simulink library "see_saw_mario"  (R2013b)
settings: Solver=ode45  StartTime=0.0  StopTime=10.0  RelTol=1e-3
undefined symbols (not defined in the file): DiscIntNeverNeededParam, K, R
libraries: legonxtlib x7, simulink x4, see_saw_mario x2
settings Model: Creator=mbiesiad  LastModifiedBy=pvinnako

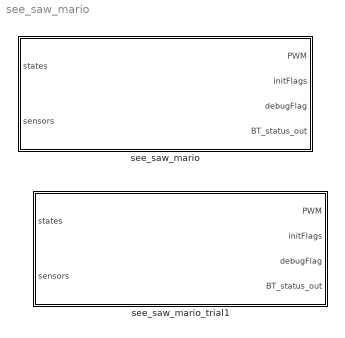
== system see_saw_mario ==
  see_saw_mario : Stateflow chart  TreatAsAtomicUnit=on
  see_saw_mario_trial1 : Stateflow chart  TreatAsAtomicUnit=on

== system see_saw_mario/see_saw_mario/see_saw_mode.DispVar ==
  Var : Inport  OutDataTypeStr=single  PortDimensions=1
  f : TriggerPort  TriggerType=function-call
      settings: CopyFcn=Stateflow.SLINSF.SimulinkMan.removeBlockPreDeleteFcn  PreDeleteFcn=Stateflow.SLINSF.SimulinkMan.unsafePredeleteFcn
  Gain : Gain  Gain=100
  LCD : legonxtlib/LCD  slcdStr=Light  slcdLine=2  slcdFormat=Decimal
  wires:
  Gain/1 -> LCD/1
  Var/1 -> Gain/1

== system see_saw_mario/see_saw_mario/see_saw_mode.Speak ==
  f : TriggerPort  TriggerType=function-call
      settings: CopyFcn=Stateflow.SLINSF.SimulinkMan.removeBlockPreDeleteFcn  PreDeleteFcn=Stateflow.SLINSF.SimulinkMan.unsafePredeleteFcn
  Constant : Constant  Value=50
  Speaker : legonxtlib/Speaker  sinputMode=Volume only  sspeakerFreq=800  sspeakerVolume=50  sspeakerDuration=100
  wires:
  Constant/1 -> Speaker/1

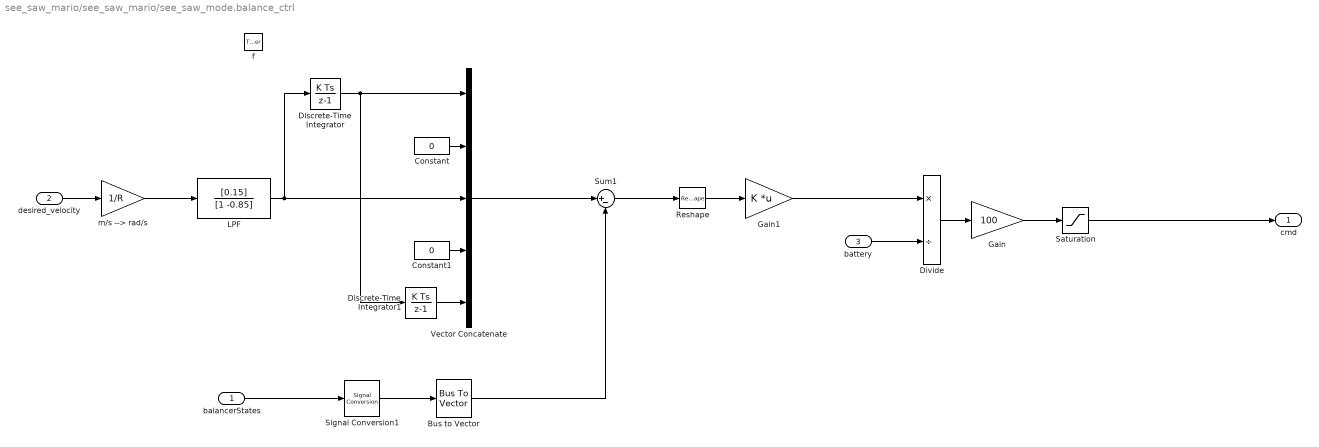
== system see_saw_mario/see_saw_mario/see_saw_mode.balance_ctrl ==
  balancerStates : Inport  OutDataTypeStr=Bus: Balancer_States_Bus  PortDimensions=1
  desired_velocity : Inport  Port=2  OutDataTypeStr=single  PortDimensions=1  BusOutputAsStruct=on
  battery : Inport  Port=3  OutDataTypeStr=double  PortDimensions=1
  f : TriggerPort  TriggerType=function-call
      settings: CopyFcn=Stateflow.SLINSF.SimulinkMan.removeBlockPreDeleteFcn  PreDeleteFcn=Stateflow.SLINSF.SimulinkMan.unsafePredeleteFcn
  Bus to Vector : BusToVector
  Constant : Constant  Value=0  OutDataTypeStr=single
  Constant1 : Constant  Value=0  OutDataTypeStr=single
  Discrete-Time Integrator : DiscreteIntegrator  SampleTime=-1  ICPrevOutput=DiscIntNeverNeededParam  ICPrevScaledInput=DiscIntNeverNeededParam
  Discrete-Time Integrator1 : DiscreteIntegrator  SampleTime=-1  ICPrevOutput=DiscIntNeverNeededParam  ICPrevScaledInput=DiscIntNeverNeededParam
  Divide : Product  Inputs=*/
  Gain : Gain  Gain=100
  Gain1 : Gain  Gain=K  Multiplication=Matrix(K*u)
  LPF : DiscreteFilter  Numerator=[0.15]  Denominator=[1 -0.85]
  Reshape : Reshape  OutputDimensionality=Column vector (2-D)
  Saturation : Saturate  UpperLimit=100  LowerLimit=-100  OutDataTypeStr=single
  Signal Conversion1 : SignalConversion  ConversionOutput=Virtual bus
  Sum1 : Sum  Inputs=|+-
  Vector Concatenate : Concatenate  NumInputs=5
  m/s --> rad/s : Gain  Gain=1/R
  cmd : Outport  OutDataTypeStr=single  PortDimensions=1  InitialOutput=0
  wires:
  Discrete-Time Integrator1/1 -> Vector Concatenate/5
  Discrete-Time Integrator/1 -> Vector Concatenate/1, Discrete-Time Integrator1/1
  Constant1/1 -> Vector Concatenate/4
  LPF/1 -> Vector Concatenate/3, Discrete-Time Integrator/1
  Constant/1 -> Vector Concatenate/2
  m/s --> rad/s/1 -> LPF/1
  Signal Conversion1/1 -> Bus to Vector/1
  Divide/1 -> Gain/1
  Gain/1 -> Saturation/1
  Gain1/1 -> Divide/1
  Saturation/1 -> cmd/1
  battery/1 -> Divide/2
  Vector Concatenate/1 -> Sum1/1
  balancerStates/1 -> Signal Conversion1/1
  Bus to Vector/1 -> Sum1/2
  desired_velocity/1 -> m/s --> rad/s/1
  Sum1/1 -> Reshape/1
  Reshape/1 -> Gain1/1

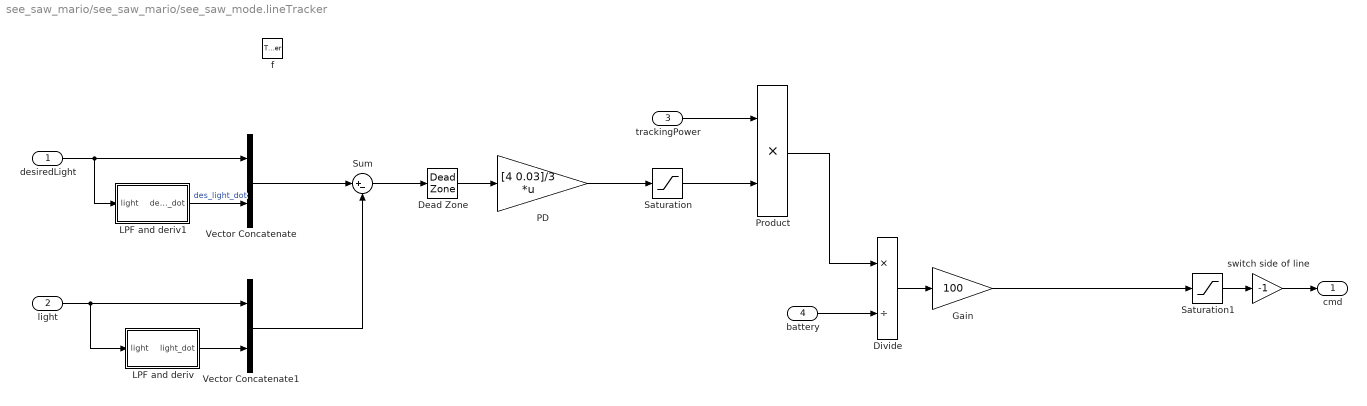
== system see_saw_mario/see_saw_mario/see_saw_mode.lineTracker ==
  desiredLight : Inport  OutDataTypeStr=single  PortDimensions=1
  light : Inport  Port=2  OutDataTypeStr=single  PortDimensions=1
  trackingPower : Inport  Port=3  OutDataTypeStr=single  PortDimensions=1
  battery : Inport  Port=4  OutDataTypeStr=double  PortDimensions=1
  f : TriggerPort  TriggerType=function-call
      settings: CopyFcn=Stateflow.SLINSF.SimulinkMan.removeBlockPreDeleteFcn  PreDeleteFcn=Stateflow.SLINSF.SimulinkMan.unsafePredeleteFcn
  Dead Zone : DeadZone  LowerValue=-0.02  UpperValue=0.02  SaturateOnIntegerOverflow=on
  Divide : Product  Inputs=*/
  Gain : Gain  Gain=100
  LPF and deriv : Subsystem
  LPF and deriv1 : Subsystem
  PD : Gain  Gain="[4  0.03]/3"  Multiplication=Matrix(K*u)
  Product : Product
  Saturation : Saturate  UpperLimit=6  LowerLimit=-6
  Saturation1 : Saturate  UpperLimit=100  LowerLimit=-100  OutDataTypeStr=single
  Sum : Sum  Inputs=|+-
  Vector Concatenate : Concatenate
  Vector Concatenate1 : Concatenate
  switch side of line : Gain  Gain=-1
  cmd : Outport  OutDataTypeStr=single  PortDimensions=1
  wires:
  Divide/1 -> Gain/1
  Gain/1 -> Saturation1/1
  battery/1 -> Divide/2
  Saturation1/1 -> switch side of line/1
  Product/1 -> Divide/1
  trackingPower/1 -> Product/1
  Saturation/1 -> Product/2
  PD/1 -> Saturation/1
  Dead Zone/1 -> PD/1
  Sum/1 -> Dead Zone/1
  Vector Concatenate1/1 -> Sum/2
  Vector Concatenate/1 -> Sum/1
  light/1 -> Vector Concatenate1/1, LPF and deriv/1(light)
  LPF and deriv/1(light_dot) -> Vector Concatenate1/2
  LPF and deriv1/1(des_light_dot) -> Vector Concatenate/2  "des_light_dot"
  desiredLight/1 -> LPF and deriv1/1(light), Vector Concatenate/1
  switch side of line/1 -> cmd/1

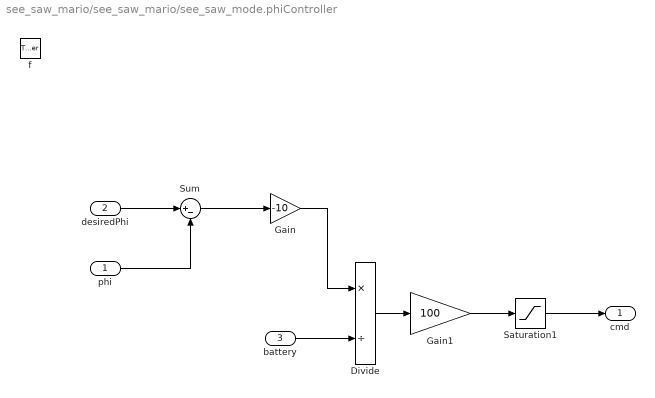
== system see_saw_mario/see_saw_mario/see_saw_mode.phiController ==
  phi : Inport  OutDataTypeStr=single  PortDimensions=1
  desiredPhi : Inport  Port=2  OutDataTypeStr=single  PortDimensions=1
  battery : Inport  Port=3  OutDataTypeStr=double  PortDimensions=1
  f : TriggerPort  TriggerType=function-call
      settings: CopyFcn=Stateflow.SLINSF.SimulinkMan.removeBlockPreDeleteFcn  PreDeleteFcn=Stateflow.SLINSF.SimulinkMan.unsafePredeleteFcn
  Divide : Product  Inputs=*/
  Gain : Gain  Gain=-10
  Gain1 : Gain  Gain=100
  Saturation1 : Saturate  UpperLimit=100  LowerLimit=-100  OutDataTypeStr=single
  Sum : Sum  Inputs=|+-
  cmd : Outport
  wires:
  Saturation1/1 -> cmd/1
  Gain/1 -> Divide/1
  Divide/1 -> Gain1/1
  Gain1/1 -> Saturation1/1
  battery/1 -> Divide/2
  Sum/1 -> Gain/1
  phi/1 -> Sum/2
  desiredPhi/1 -> Sum/1

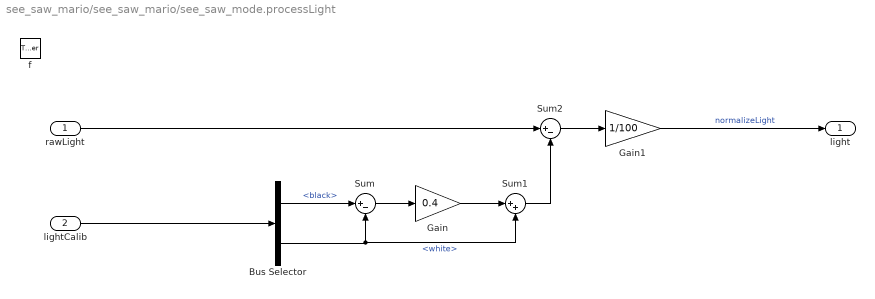
== system see_saw_mario/see_saw_mario/see_saw_mode.processLight ==
  rawLight : Inport  OutDataTypeStr=single  PortDimensions=1
  lightCalib : Inport  Port=2  OutDataTypeStr=Bus: Light_Bus  PortDimensions=1
  f : TriggerPort  TriggerType=function-call
      settings: CopyFcn=Stateflow.SLINSF.SimulinkMan.removeBlockPreDeleteFcn  PreDeleteFcn=Stateflow.SLINSF.SimulinkMan.unsafePredeleteFcn
  Bus Selector : BusSelector  OutputSignals=black,white
  Gain : Gain  Gain=0.4
  Gain1 : Gain  Gain=1/100
  Sum : Sum  Inputs=|+-
  Sum1 : Sum  Inputs=|++
  Sum2 : Sum  Inputs=|+-
  light : Outport
  wires:
  Gain1/1 -> light/1  "normalizeLight"
  Sum2/1 -> Gain1/1
  Sum1/1 -> Sum2/2
  rawLight/1 -> Sum2/1
  Gain/1 -> Sum1/1
  Sum/1 -> Gain/1
  Bus Selector/2 -> Sum/2, Sum1/2  "<white>"
  Bus Selector/1 -> Sum/1  "<black>"
  lightCalib/1 -> Bus Selector/1

== system see_saw_mario/see_saw_mario/see_saw_mode.tail_controller ==
  note: Could be improved, PI for example
  current : Inport  OutDataTypeStr=single  PortDimensions=1
  desired : Inport  Port=2  OutDataTypeStr=single  PortDimensions=1
  f : TriggerPort  TriggerType=function-call
      settings: CopyFcn=Stateflow.SLINSF.SimulinkMan.removeBlockPreDeleteFcn  PreDeleteFcn=Stateflow.SLINSF.SimulinkMan.unsafePredeleteFcn
  Gain : Gain  Gain=250
  Saturation : Saturate  UpperLimit=100  LowerLimit=-100  OutDataTypeStr=single
  Sum : Sum  Inputs=|+-
  cmd : Outport  OutDataTypeStr=single  PortDimensions=1  InitialOutput=0
  wires:
  Saturation/1 -> cmd/1
  Gain/1 -> Saturation/1
  desired/1 -> Sum/1
  current/1 -> Sum/2
  Sum/1 -> Gain/1

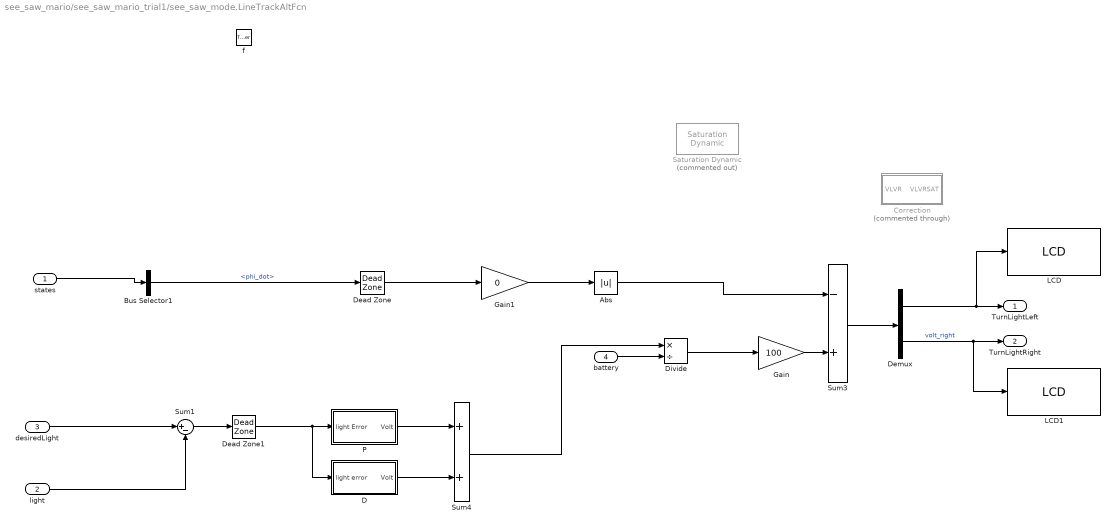
== system see_saw_mario/see_saw_mario_trial1/see_saw_mode.LineTrackAltFcn ==
  states : Inport  OutDataTypeStr=Bus: States_Bus  PortDimensions=1
  light : Inport  Port=2  OutDataTypeStr=single  PortDimensions=1
  desiredLight : Inport  Port=3  OutDataTypeStr=single  PortDimensions=1
  battery : Inport  Port=4  OutDataTypeStr=single  PortDimensions=1
  f : TriggerPort  TriggerType=function-call
      settings: CopyFcn=Stateflow.SLINSF.SimulinkMan.removeBlockPreDeleteFcn  PreDeleteFcn=Stateflow.SLINSF.SimulinkMan.unsafePredeleteFcn
  Abs : Abs
  Bus Selector1 : BusSelector  OutputSignals=phi_dot
  Correction : Subsystem  Commented=through
  D : Subsystem
  Dead Zone : DeadZone  LowerValue=-3  UpperValue=3  SaturateOnIntegerOverflow=on
  Dead Zone1 : DeadZone  LowerValue=0  UpperValue=0  SaturateOnIntegerOverflow=on
  Demux : Demux  Outputs=2
  Divide : Product  Inputs=*/
  Gain : Gain  Gain=100
  Gain1 : Gain  Gain=0
  LCD : legonxtlib/LCD  slcdStr=TurnL  slcdLine=5  slcdFormat=Decimal
  LCD1 : legonxtlib/LCD  slcdStr=TurnR  slcdLine=6  slcdFormat=Decimal
  P : Subsystem
  Saturation Dynamic : simulink/Discontinuities/Saturation Dynamic  Commented=on  OutMin=[]  OutMax=[]  OutDataTypeStr=Inherit: Same as second input  OutDataType=fixdt(1, 16)  OutScaling=2^-10  DoSatur=off
  Sum1 : Sum  Inputs=|+-
  Sum3 : Sum  Inputs=-+
  Sum4 : Sum
  TurnLightLeft : Outport  OutDataTypeStr=single  InitialOutput=0
  TurnLightRight : Outport  Port=2  OutDataTypeStr=single  InitialOutput=0
  wires:
  Dead Zone1/1 -> D/1(light error), P/1(light Error)
  Dead Zone/1 -> Gain1/1
  Demux/2 -> LCD1/1, TurnLightRight/1  "volt_right"
  Demux/1 -> LCD/1, TurnLightLeft/1
  light/1 -> Sum1/2
  Sum1/1 -> Dead Zone1/1
  states/1 -> Bus Selector1/1
  desiredLight/1 -> Sum1/1
  P/1(Volt) -> Sum4/1
  D/1(Volt) -> Sum4/2
  Gain/1 -> Sum3/2
  Abs/1 -> Sum3/1
  Gain1/1 -> Abs/1
  Bus Selector1/1 -> Dead Zone/1  "<phi_dot>"
  Sum3/1 -> Demux/1
  battery/1 -> Divide/2
  Divide/1 -> Gain/1
  Sum4/1 -> Divide/1

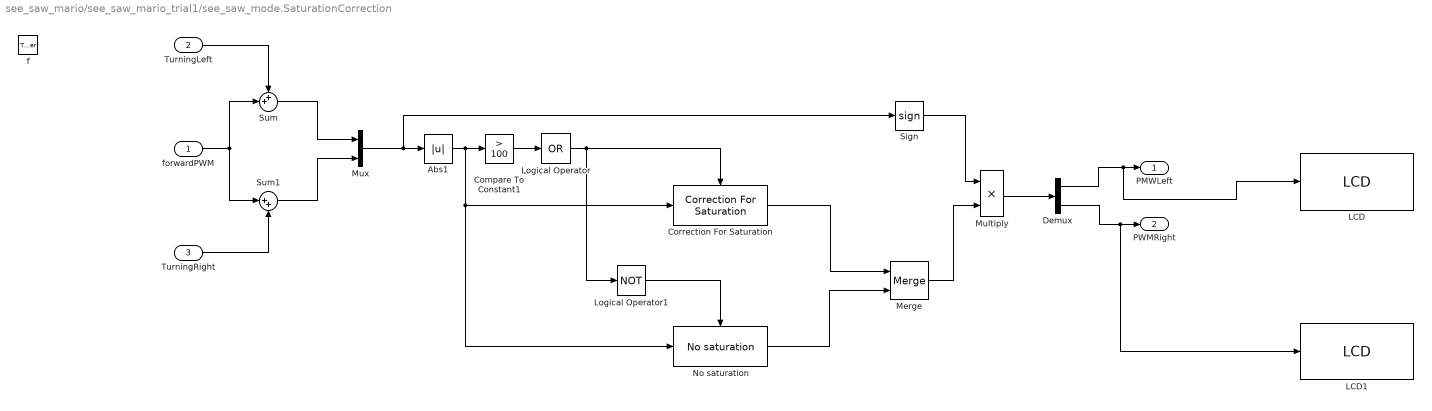
== system see_saw_mario/see_saw_mario_trial1/see_saw_mode.SaturationCorrection ==
  forwardPWM : Inport  OutDataTypeStr=single  PortDimensions=1
  TurningLeft : Inport  Port=2  OutDataTypeStr=single  PortDimensions=1
  TurningRight : Inport  Port=3  OutDataTypeStr=single  PortDimensions=1
  f : TriggerPort  TriggerType=function-call
      settings: CopyFcn=Stateflow.SLINSF.SimulinkMan.removeBlockPreDeleteFcn  PreDeleteFcn=Stateflow.SLINSF.SimulinkMan.unsafePredeleteFcn
  Abs1 : Abs
  Compare To Constant1 : simulink/Logic and Bit Operations/Compare To Constant  relop=>  const=100  OutDataTypeStr=boolean
  Correction For Saturation : see_saw_mario/see_saw_mario/see_saw_mode.LineTrackAltFcn/Correction/Correction For Saturation
  Demux : Demux  Outputs=2
  LCD : legonxtlib/LCD  slcdStr=VL  slcdLine=3  slcdFormat=Decimal
  LCD1 : legonxtlib/LCD  slcdStr=VR  slcdLine=4  slcdFormat=Decimal
  Logical Operator : Logic  Operator=OR  Inputs=1  AllPortsSameDT=off  OutDataTypeStr=boolean
  Logical Operator1 : Logic  Operator=NOT  Inputs=1  AllPortsSameDT=off  OutDataTypeStr=boolean
  Merge : Merge
  Multiply : Product  Inputs=**
  Mux : Mux  Inputs=2
  No saturation : see_saw_mario/see_saw_mario/see_saw_mode.LineTrackAltFcn/Correction/No saturation
  Sign : Signum
  Sum : Sum  Inputs=++|
  Sum1 : Sum  Inputs=|++
  PMWLeft : Outport  OutDataTypeStr=single  PortDimensions=1
  PWMRight : Outport  Port=2  OutDataTypeStr=single  PortDimensions=1
  wires:
  Mux/1 -> Sign/1, Abs1/1
  Abs1/1 -> No saturation/1, Correction For Saturation/1, Compare To Constant1/1
  Compare To Constant1/1 -> Logical Operator/1
  Logical Operator/1 -> Logical Operator1/1, Correction For Saturation/Enable
  Logical Operator1/1 -> No saturation/Enable
  Correction For Saturation/1 -> Merge/1
  No saturation/1 -> Merge/2
  Merge/1 -> Multiply/2
  Sign/1 -> Multiply/1
  Multiply/1 -> Demux/1
  forwardPWM/1 -> Sum1/1, Sum/2
  TurningLeft/1 -> Sum/1
  TurningRight/1 -> Sum1/2
  Sum/1 -> Mux/1
  Sum1/1 -> Mux/2
  Demux/1 -> LCD/1, PMWLeft/1
  Demux/2 -> LCD1/1, PWMRight/1

== system see_saw_mario/see_saw_mario_trial1/see_saw_mode.Speak ==
  f : TriggerPort  TriggerType=function-call
      settings: CopyFcn=Stateflow.SLINSF.SimulinkMan.removeBlockPreDeleteFcn  PreDeleteFcn=Stateflow.SLINSF.SimulinkMan.unsafePredeleteFcn
  Constant : Constant  Value=50
  Speaker : legonxtlib/Speaker  sinputMode=Volume only  sspeakerFreq=800  sspeakerVolume=50  sspeakerDuration=100
  wires:
  Constant/1 -> Speaker/1

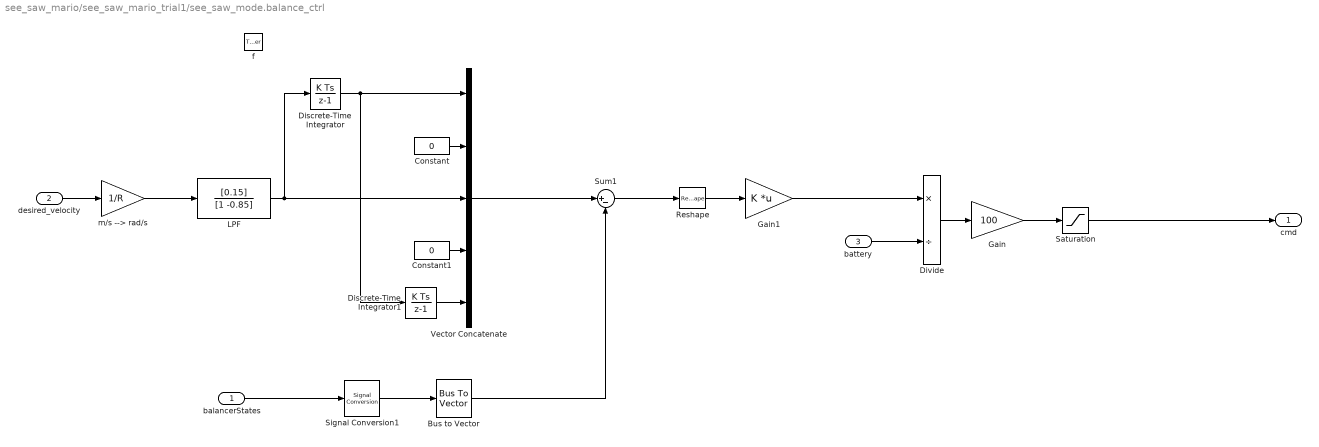
== system see_saw_mario/see_saw_mario_trial1/see_saw_mode.balance_ctrl ==
  balancerStates : Inport  OutDataTypeStr=Bus: Balancer_States_Bus  PortDimensions=1
  desired_velocity : Inport  Port=2  OutDataTypeStr=single  PortDimensions=1  BusOutputAsStruct=on
  battery : Inport  Port=3  OutDataTypeStr=double  PortDimensions=1
  f : TriggerPort  TriggerType=function-call
      settings: CopyFcn=Stateflow.SLINSF.SimulinkMan.removeBlockPreDeleteFcn  PreDeleteFcn=Stateflow.SLINSF.SimulinkMan.unsafePredeleteFcn
  Bus to Vector : BusToVector
  Constant : Constant  Value=0  OutDataTypeStr=single
  Constant1 : Constant  Value=0  OutDataTypeStr=single
  Discrete-Time Integrator : DiscreteIntegrator  SampleTime=-1  ICPrevOutput=DiscIntNeverNeededParam  ICPrevScaledInput=DiscIntNeverNeededParam
  Discrete-Time Integrator1 : DiscreteIntegrator  SampleTime=-1  ICPrevOutput=DiscIntNeverNeededParam  ICPrevScaledInput=DiscIntNeverNeededParam
  Divide : Product  Inputs=*/
  Gain : Gain  Gain=100
  Gain1 : Gain  Gain=K  Multiplication=Matrix(K*u)
  LPF : DiscreteFilter  Numerator=[0.15]  Denominator=[1 -0.85]
  Reshape : Reshape  OutputDimensionality=Column vector (2-D)
  Saturation : Saturate  UpperLimit=100  LowerLimit=-100  OutDataTypeStr=single
  Signal Conversion1 : SignalConversion  ConversionOutput=Virtual bus
  Sum1 : Sum  Inputs=|+-
  Vector Concatenate : Concatenate  NumInputs=5
  m/s --> rad/s : Gain  Gain=1/R
  cmd : Outport  OutDataTypeStr=single  PortDimensions=1  InitialOutput=0
  wires:
  Reshape/1 -> Gain1/1
  Sum1/1 -> Reshape/1
  desired_velocity/1 -> m/s --> rad/s/1
  Bus to Vector/1 -> Sum1/2
  balancerStates/1 -> Signal Conversion1/1
  Vector Concatenate/1 -> Sum1/1
  battery/1 -> Divide/2
  Saturation/1 -> cmd/1
  Gain1/1 -> Divide/1
  Gain/1 -> Saturation/1
  Divide/1 -> Gain/1
  Signal Conversion1/1 -> Bus to Vector/1
  m/s --> rad/s/1 -> LPF/1
  Constant/1 -> Vector Concatenate/2
  LPF/1 -> Discrete-Time Integrator/1, Vector Concatenate/3
  Constant1/1 -> Vector Concatenate/4
  Discrete-Time Integrator/1 -> Discrete-Time Integrator1/1, Vector Concatenate/1
  Discrete-Time Integrator1/1 -> Vector Concatenate/5

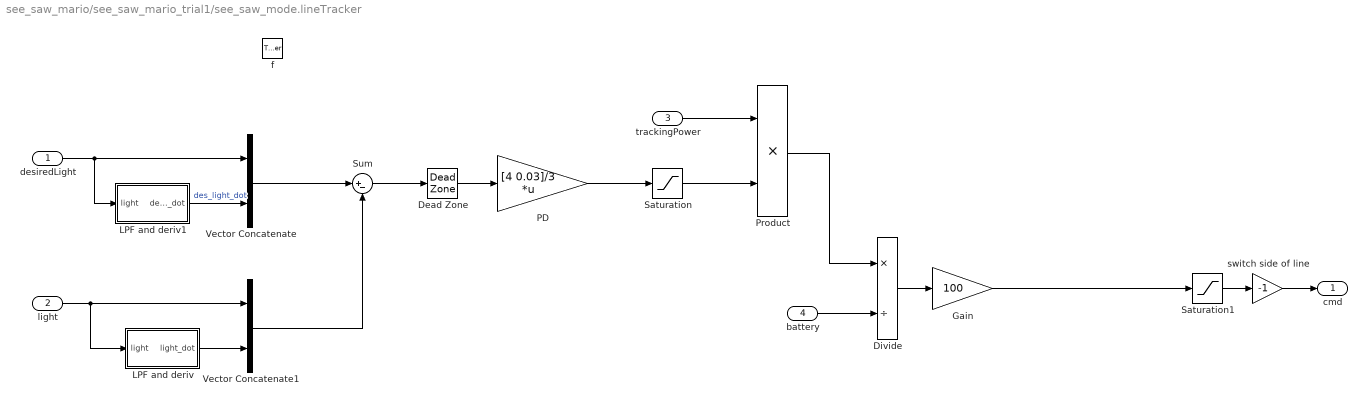
== system see_saw_mario/see_saw_mario_trial1/see_saw_mode.lineTracker ==
  desiredLight : Inport  OutDataTypeStr=single  PortDimensions=1
  light : Inport  Port=2  OutDataTypeStr=single  PortDimensions=1
  trackingPower : Inport  Port=3  OutDataTypeStr=single  PortDimensions=1
  battery : Inport  Port=4  OutDataTypeStr=double  PortDimensions=1
  f : TriggerPort  TriggerType=function-call
      settings: CopyFcn=Stateflow.SLINSF.SimulinkMan.removeBlockPreDeleteFcn  PreDeleteFcn=Stateflow.SLINSF.SimulinkMan.unsafePredeleteFcn
  Dead Zone : DeadZone  LowerValue=-0.02  UpperValue=0.02  SaturateOnIntegerOverflow=on
  Divide : Product  Inputs=*/
  Gain : Gain  Gain=100
  LPF and deriv : Subsystem
  LPF and deriv1 : Subsystem
  PD : Gain  Gain="[4  0.03]/3"  Multiplication=Matrix(K*u)
  Product : Product
  Saturation : Saturate  UpperLimit=6  LowerLimit=-6
  Saturation1 : Saturate  UpperLimit=100  LowerLimit=-100  OutDataTypeStr=single
  Sum : Sum  Inputs=|+-
  Vector Concatenate : Concatenate
  Vector Concatenate1 : Concatenate
  switch side of line : Gain  Gain=-1
  cmd : Outport  OutDataTypeStr=single  PortDimensions=1
  wires:
  switch side of line/1 -> cmd/1
  desiredLight/1 -> Vector Concatenate/1, LPF and deriv1/1(light)
  LPF and deriv1/1(des_light_dot) -> Vector Concatenate/2  "des_light_dot"
  LPF and deriv/1(light_dot) -> Vector Concatenate1/2
  light/1 -> LPF and deriv/1(light), Vector Concatenate1/1
  Vector Concatenate/1 -> Sum/1
  Vector Concatenate1/1 -> Sum/2
  Sum/1 -> Dead Zone/1
  Dead Zone/1 -> PD/1
  PD/1 -> Saturation/1
  Saturation/1 -> Product/2
  trackingPower/1 -> Product/1
  Product/1 -> Divide/1
  Saturation1/1 -> switch side of line/1
  battery/1 -> Divide/2
  Gain/1 -> Saturation1/1
  Divide/1 -> Gain/1

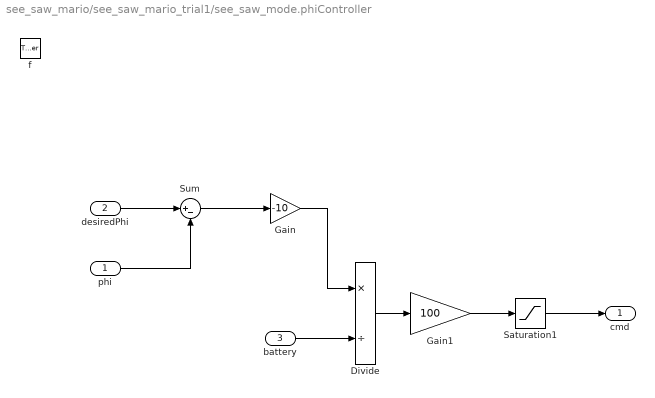
== system see_saw_mario/see_saw_mario_trial1/see_saw_mode.phiController ==
  phi : Inport  OutDataTypeStr=single  PortDimensions=1
  desiredPhi : Inport  Port=2  OutDataTypeStr=single  PortDimensions=1
  battery : Inport  Port=3  OutDataTypeStr=double  PortDimensions=1
  f : TriggerPort  TriggerType=function-call
      settings: CopyFcn=Stateflow.SLINSF.SimulinkMan.removeBlockPreDeleteFcn  PreDeleteFcn=Stateflow.SLINSF.SimulinkMan.unsafePredeleteFcn
  Divide : Product  Inputs=*/
  Gain : Gain  Gain=-10
  Gain1 : Gain  Gain=100
  Saturation1 : Saturate  UpperLimit=100  LowerLimit=-100  OutDataTypeStr=single
  Sum : Sum  Inputs=|+-
  cmd : Outport
  wires:
  desiredPhi/1 -> Sum/1
  phi/1 -> Sum/2
  Sum/1 -> Gain/1
  battery/1 -> Divide/2
  Gain1/1 -> Saturation1/1
  Divide/1 -> Gain1/1
  Gain/1 -> Divide/1
  Saturation1/1 -> cmd/1

== system see_saw_mario/see_saw_mario_trial1/see_saw_mode.processLight ==
  rawLight : Inport  OutDataTypeStr=single  PortDimensions=1
  lightCalib : Inport  Port=2  OutDataTypeStr=Bus: Light_Bus  PortDimensions=1
  f : TriggerPort  TriggerType=function-call
      settings: CopyFcn=Stateflow.SLINSF.SimulinkMan.removeBlockPreDeleteFcn  PreDeleteFcn=Stateflow.SLINSF.SimulinkMan.unsafePredeleteFcn
  Bus Selector : BusSelector  OutputSignals=black,white
  Gain : Gain  Gain=0.3
  Gain1 : Gain  Gain=1/100
  Sum : Sum  Inputs=|+-
  Sum1 : Sum  Inputs=|++
  Sum2 : Sum  Inputs=|+-
  light : Outport
  wires:
  lightCalib/1 -> Bus Selector/1
  Bus Selector/1 -> Sum/1  "<black>"
  Bus Selector/2 -> Sum1/2, Sum/2  "<white>"
  Sum/1 -> Gain/1
  Gain/1 -> Sum1/1
  rawLight/1 -> Sum2/1
  Sum1/1 -> Sum2/2
  Sum2/1 -> Gain1/1
  Gain1/1 -> light/1  "normalizeLight"

== system see_saw_mario/see_saw_mario_trial1/see_saw_mode.tail_controller ==
  note: Could be improved, PI for example
  current : Inport  OutDataTypeStr=single  PortDimensions=1
  desired : Inport  Port=2  OutDataTypeStr=single  PortDimensions=1
  f : TriggerPort  TriggerType=function-call
      settings: CopyFcn=Stateflow.SLINSF.SimulinkMan.removeBlockPreDeleteFcn  PreDeleteFcn=Stateflow.SLINSF.SimulinkMan.unsafePredeleteFcn
  Gain : Gain  Gain=250
  Saturation : Saturate  UpperLimit=100  LowerLimit=-100  OutDataTypeStr=single
  Sum : Sum  Inputs=|+-
  cmd : Outport  OutDataTypeStr=single  PortDimensions=1  InitialOutput=0
  wires:
  Sum/1 -> Gain/1
  current/1 -> Sum/2
  desired/1 -> Sum/1
  Gain/1 -> Saturation/1
  Saturation/1 -> cmd/1

== system see_saw_mario/see_saw_mario/see_saw_mode.lineTracker/LPF and deriv ==
  light : Inport
  Discrete Filter : DiscreteFilter  Numerator=[0.05]  Denominator=[1 -0.95]
  Gain : Gain  Gain=1/0.004
  Sum3 : Sum  Inputs=+-
  Unit Delay : UnitDelay  SampleTime=-1
  light_dot : Outport
  wires:
  Unit Delay/1 -> Sum3/2
  Gain/1 -> Unit Delay/1, Sum3/1
  Sum3/1 -> light_dot/1  "light_dot"
  Discrete Filter/1 -> Gain/1
  light/1 -> Discrete Filter/1

== system see_saw_mario/see_saw_mario/see_saw_mode.lineTracker/LPF and deriv1 ==
  light : Inport
  Discrete Filter : DiscreteFilter  Numerator=[0.05]  Denominator=[1 -0.95]
  Gain : Gain  Gain=1/0.004
  Sum3 : Sum  Inputs=+-
  Unit Delay : UnitDelay  SampleTime=-1
  des_light_dot : Outport
  wires:
  light/1 -> Discrete Filter/1
  Discrete Filter/1 -> Gain/1
  Sum3/1 -> des_light_dot/1  "des_light_dot"
  Gain/1 -> Sum3/1, Unit Delay/1
  Unit Delay/1 -> Sum3/2

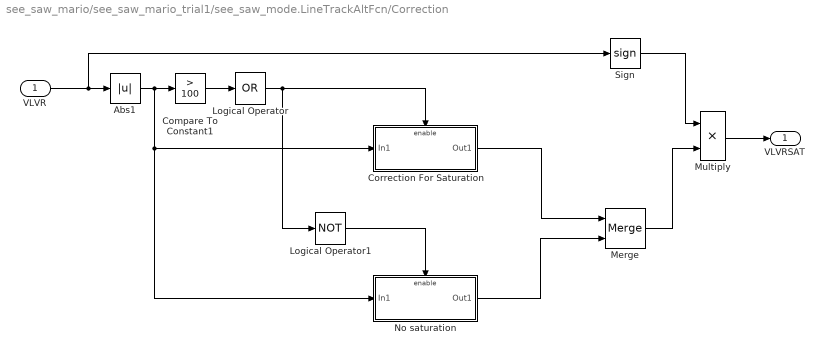
== system see_saw_mario/see_saw_mario_trial1/see_saw_mode.LineTrackAltFcn/Correction ==
  VLVR : Inport
  Abs1 : Abs
  Compare To Constant1 : simulink/Logic and Bit Operations/Compare To Constant  relop=>  const=100  OutDataTypeStr=boolean
  Correction For Saturation : Subsystem  TreatAsAtomicUnit=on
  Logical Operator : Logic  Operator=OR  Inputs=1  AllPortsSameDT=off  OutDataTypeStr=boolean
  Logical Operator1 : Logic  Operator=NOT  Inputs=1  AllPortsSameDT=off  OutDataTypeStr=boolean
  Merge : Merge
  Multiply : Product  Inputs=**
  No saturation : Subsystem  TreatAsAtomicUnit=on
  Sign : Signum
  VLVRSAT : Outport
  wires:
  VLVR/1 -> Sign/1, Abs1/1
  Abs1/1 -> No saturation/1(In1), Correction For Saturation/1(In1), Compare To Constant1/1
  Compare To Constant1/1 -> Logical Operator/1
  Logical Operator/1 -> Logical Operator1/1, Correction For Saturation/Enable
  Logical Operator1/1 -> No saturation/Enable
  Correction For Saturation/1(Out1) -> Merge/1
  No saturation/1(Out1) -> Merge/2
  Merge/1 -> Multiply/2
  Sign/1 -> Multiply/1
  Multiply/1 -> VLVRSAT/1

== system see_saw_mario/see_saw_mario_trial1/see_saw_mode.LineTrackAltFcn/D ==
  light error : Inport
  Abs1 : Abs
  Constant4 : Constant  Value=[3 0]  OutDataTypeStr=single
  Constant5 : Constant  Value=[0 1]  OutDataTypeStr=single
  Discrete Derivative1 : simulink/Discrete/Discrete Derivative  gainval=1.0  ICPrevScaledInput=0.0  InputProcessing=Inherited  OutMin=[]  OutMax=[]  OutDataTypeStr=single  OutputDataTypeScalingMode=single  OutDataType=fixdt(1, 16)  OutScaling=2^-10  DoSatur=off
  Gain2 : Gain  Gain=0.002*10*3
  Low Pass Filter1 : DiscreteFilter  Numerator=[.2]  Denominator=[1 -0.8]
  Product1 : Product  RndMeth=Zero
  Switch1 : Switch
  Volt : Outport
  wires:
  light error/1 -> Low Pass Filter1/1
  Low Pass Filter1/1 -> Discrete Derivative1/1
  Abs1/1 -> Gain2/1
  Constant5/1 -> Switch1/3
  Constant4/1 -> Switch1/1
  Discrete Derivative1/1 -> Switch1/2, Abs1/1
  Switch1/1 -> Product1/1
  Gain2/1 -> Product1/2
  Product1/1 -> Volt/1

== system see_saw_mario/see_saw_mario_trial1/see_saw_mode.LineTrackAltFcn/P ==
  light Error : Inport
  Abs : Abs
  Constant2 : Constant  Value=[3 0]  OutDataTypeStr=single
  Constant3 : Constant  Value=[0 1]  OutDataTypeStr=single
  Gain4 : Gain  Gain=0.05*10*3
  Product : Product  RndMeth=Zero
  Switch : Switch
  Volt : Outport
  wires:
  light Error/1 -> Abs/1, Switch/2
  Switch/1 -> Product/1
  Constant3/1 -> Switch/3
  Constant2/1 -> Switch/1
  Abs/1 -> Gain4/1
  Gain4/1 -> Product/2
  Product/1 -> Volt/1

== system see_saw_mario/see_saw_mario_trial1/see_saw_mode.lineTracker/LPF and deriv ==
  light : Inport
  Discrete Filter : DiscreteFilter  Numerator=[0.05]  Denominator=[1 -0.95]
  Gain : Gain  Gain=1/0.004
  Sum3 : Sum  Inputs=+-
  Unit Delay : UnitDelay  SampleTime=-1
  light_dot : Outport
  wires:
  light/1 -> Discrete Filter/1
  Discrete Filter/1 -> Gain/1
  Sum3/1 -> light_dot/1  "light_dot"
  Gain/1 -> Sum3/1, Unit Delay/1
  Unit Delay/1 -> Sum3/2

== system see_saw_mario/see_saw_mario_trial1/see_saw_mode.lineTracker/LPF and deriv1 ==
  light : Inport
  Discrete Filter : DiscreteFilter  Numerator=[0.05]  Denominator=[1 -0.95]
  Gain : Gain  Gain=1/0.004
  Sum3 : Sum  Inputs=+-
  Unit Delay : UnitDelay  SampleTime=-1
  des_light_dot : Outport
  wires:
  Unit Delay/1 -> Sum3/2
  Gain/1 -> Unit Delay/1, Sum3/1
  Sum3/1 -> des_light_dot/1  "des_light_dot"
  Discrete Filter/1 -> Gain/1
  light/1 -> Discrete Filter/1

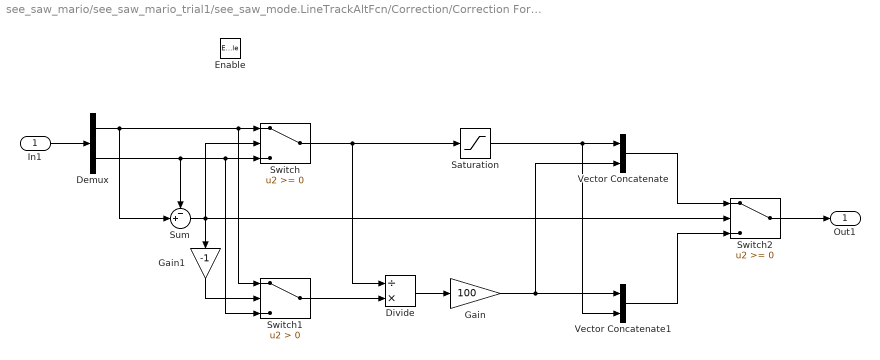
== system see_saw_mario/see_saw_mario_trial1/see_saw_mode.LineTrackAltFcn/Correction/Correction For Saturation ==
  In1 : Inport
  Enable : EnablePort
  Demux : Demux  Outputs=2
  Divide : Product  Inputs=/*
  Gain : Gain  Gain=100
  Gain1 : Gain  Gain=-1
  Saturation : Saturate  UpperLimit=100  LowerLimit=-100
  Sum : Sum  Inputs=-+|
  Switch : Switch
  Switch1 : Switch  Criteria=u2 > Threshold
  Switch2 : Switch
  Vector Concatenate : Concatenate
  Vector Concatenate1 : Concatenate
  Out1 : Outport
  wires:
  In1/1 -> Demux/1
  Demux/1 -> Sum/2, Switch1/1, Switch/1
  Demux/2 -> Sum/1, Switch1/3, Switch/3
  Sum/1 -> Gain1/1, Switch2/2, Switch/2
  Switch/1 -> Divide/1, Saturation/1
  Saturation/1 -> Vector Concatenate1/2, Vector Concatenate/1
  Switch1/1 -> Divide/2
  Divide/1 -> Gain/1
  Gain1/1 -> Switch1/2
  Gain/1 -> Vector Concatenate/2, Vector Concatenate1/1
  Vector Concatenate/1 -> Switch2/1
  Vector Concatenate1/1 -> Switch2/3
  Switch2/1 -> Out1/1

== system see_saw_mario/see_saw_mario_trial1/see_saw_mode.LineTrackAltFcn/Correction/No saturation ==
  In1 : Inport
  Enable : EnablePort
  Out1 : Outport
  wires:
  In1/1 -> Out1/1

== stateflow chart see_saw_mario/see_saw_mario_trial1 ==
  state see_saw_mode
    entry:
    desired_tail = single(1.6);
    BT_status_out = single(0);
    during:
    normalizedLight = processLight(sensors.light,lightCalib);
    PWM.tail = tail_controller(sensors.theta_T, desired_tail);
    state Pause
      entry:
      debugFlag = uint16(601);
    state light = processLight(rawLight,lightCalib) [function]
    state StandUp
      entry: debugFlag = uint16(602);
      initFlags.theta = single(1);
      initFlags.gyroReset = single(1);
      during:
      desired_tail = desired_tail + single(0.0008);
    state Balancing
      state SeesawLogic [parallel]
        settings: executionOrder=1
        state StationnaryBalance
          entry: debugFlag = uint16(603);
          desired_tail = single(0.5);
          initFlags.theta = single(0);
          initFlags.gyroReset = single(0);
          desired_states = balancerStates_Bus0;
        state Approach
          entry: debugFlag = uint16(604);
          during:
          [turningPWML, turningPWMR] = LineTrackAltFcn(states, normalizedLight, single(0), sensors.battery);
          exit:
          turningPWM = single(0);
          state StartWalking
            entry:
            entry: debugFlag = uint16(605);
            des_vel = single(0.04);
            during:
            des_vel = des_vel+single(0.00024);
          state Walk
            entry: debugFlag = uint16(605);
          (default) -> StartWalking
          StartWalking -> Walk : [des_vel >= single(0.15)]
        state Seesaw
          state ControlledGoingUp
            entry:
            phi0 = states.phi;
            desired_phi = phi0;
            exit: turningPWM = single(0);
            state JumpOnIt
              entry:
              Speak;
              debugFlag = uint16(606);
              theta_ref = states.balancerStates.theta;
              des_vel = single(0.15);
            state GoingUP
              entry:
              debugFlag = uint16(607);
              des_vel = single(0.1);
              during:
              turningPWM = phiController(states.phi,desired_phi, sensors.battery)+...
              single(3)*lineTracker(single(0.15), normalizedLight, single(1), sensors.battery);
              exit:
              des_vel = single(0);
            state WaitForPrincess
              entry:
              debugFlag = uint16(608);
              BT_status_out = single(2);
              du:
              turningPWM = phiController(states.phi,desired_phi,sensors.battery);
            (default) -> JumpOnIt
            JumpOnIt -> GoingUP : [states.balancerStates.theta >= theta_ref+single(1.57)]
            GoingUP -> WaitForPrincess : [states.balancerStates.theta >= theta_ref + single(18)]
          state GoingDown
            during:
            turningPWM = single(-1.3)*lineTracker(single(0.3), normalizedLight, single(1), sensors.battery)+...
            single(1)*phiController(states.phi,desired_phi,sensors.battery);
            state GoingBack
              entry:
              debugFlag = uint16(609);
              des_vel = single(-0.06);
              exit:
              des_vel = single(0);
            state Pause2
              during:turningPWM = phiController(states.phi,desired_phi,sensors.battery);
            state WaitForPrincess2
              entry:
              debugFlag = uint16(610);
              BT_status_out = single(3);
              during:turningPWM = phiController(states.phi,desired_phi,sensors.battery);
            state GetOff
              entry:
              debugFlag = uint16(611);
              des_vel = single(-0.08);
              exit:
              des_vel = single(0);
            state Pause3
              during:
              turningPWM = phiController(states.phi,desired_phi,sensors.battery);
            (default) -> GoingBack
            GoingBack -> Pause2 : [states.balancerStates.theta <= theta_ref + single(5.5)]
            Pause2 -> WaitForPrincess2 : after(3,sec)
            WaitForPrincess2 -> GetOff : [sensors.BT_status_in == single(103)]
            GetOff -> Pause3 : [states.balancerStates.theta <= theta_ref - single(7)]
          state FindingLine
            en:
            turningPWM = phiController(states.phi,desired_phi,sensors.battery);
            des_vel = single(0);
            state TurnAndBackup
              entry:
              debugFlag = uint16(612);
              BT_status_out = single(4);
              du:
              desired_phi = desired_phi - single(0.003);
              des_vel = single(-0.015);
              turningPWM = phiController(states.phi,desired_phi,sensors.battery);
            state GoForwardUntilLine
              en:
              debugFlag = uint16(613)
              desired_phi = states.phi;
              du:
              turningPWM = lineTracker(single(0), normalizedLight, single(0.4), sensors.battery);
              des_vel= single(0.04);
            state BeginLineTrack
              en:
              debugFlag = uint16(614);
              des_vel =single(0.05);
              du:
              des_vel = des_vel+single(0.0004);
              turningPWM = lineTracker(single(0), normalizedLight, single(0.8), sensors.battery);
            state ConstantSpeedAlongLIne
              en:
              debugFlag = uint16(615);
              du:
              turningPWM = lineTracker(single(0), normalizedLight, single(1), sensors.battery);
            state STOP
              en:
              des_vel = single(0);
            (default) -> TurnAndBackup
            TurnAndBackup -> GoForwardUntilLine : [phi0-states.phi > single(3)]
            GoForwardUntilLine -> BeginLineTrack : [normalizedLight >= single(0.5)]
            BeginLineTrack -> ConstantSpeedAlongLIne : [des_vel >= single(0.08)]
            ConstantSpeedAlongLIne -> STOP : [false] %[states.balancerStates.theta <= theta_ref - single(2)]
          (default) -> ControlledGoingUp
          WaitForPrincess -> GoingDown : [sensors.BT_status_in == single(102)]
          Pause3 -> FindingLine : after(2,sec)
        state RaceDone
          entry: debugFlag = uint16(599);
          current_mode_status = OperationModeStatusEnum.SUCCESSFULLY_COMPLETED;
        (default) -> StationnaryBalance
        StationnaryBalance -> Approach : after(5,sec)
        Approach -> ? : [states.balancerStates.theta_dot<single(-4)  && states.theta_dot_dot < single(-60) ]{BT_status_out = single(1);}
      state After [parallel]
        during:
        forwardPWM = balance_ctrl(states.balancerStates, des_vel ,sensors.battery)
        %PWM.left = forwardPWM + turningPWM;
        %PWM.right = forwardPWM - turningPWM;
        [PWM.left, PWM.right] = SaturationCorrection(forwardPWM, turningPWML, turningPWMR)
        settings: executionOrder=2
    state [PMWLeft,PWMRight] = SaturationCorrection(forwardPWM,TurningLeft,TurningRight) [function]
    state [TurnLightLeft,TurnLightRight] = LineTrackAltFcn(states,light,desiredLight,battery) [function]
    state cmd = phiController(phi,desiredPhi,battery) [function]
    state cmd = lineTracker(desiredLight,light,trackingPower,battery) [function]
    state Speak [function]
    state cmd = tail_controller(current,desired) [function]
    state cmd = balance_ctrl(balancerStates,desired_velocity,battery) [function]
    (default) -> Pause
    Pause -> StandUp : after(1,sec)
    StandUp -> Balancing : [desired_tail >=single(2.0) && sensors.theta_T >= single(2.0)]
  data: rawLight function_input single size=1; lightCalib function_input Bus: Light_Bus size=1; light function_output; PMWLeft function_output single size=1; forwardPWM function_input single size=1; TurningLeft function_input single size=1; TurningRight function_input single size=1; PWMRight function_output single size=1; states function_input Bus: States_Bus size=1; TurnLightLeft function_output single; TurnLightRight function_output single; light function_input single size=1; desiredLight function_input single size=1; battery function_input single size=1; cmd function_output; phi function_input single size=1; desiredPhi function_input single size=1; battery function_input double size=1; cmd function_output single size=1; desiredLight function_input single size=1; light function_input single size=1; trackingPower function_input single size=1; battery function_input double size=1; current function_input single size=1; desired function_input single size=1; cmd function_output single size=1; balancerStates function_input Bus: Balancer_States_Bus size=1; desired_velocity function_input single size=1; battery function_input double size=1; cmd function_output single size=1; states input Bus: States_Bus size=1; sensors input Bus: Sensors_Bus size=1; PWM output Bus: PWM_bus size=1; initFlags output Bus: Init_Bus size=1; debugFlag output uint16 size=1; desired_states local Bus: Balancer_States_Bus size=1; desired_tail local single size=1; current_mode_status data_store_memory; balancerStates_Bus0 parameter Bus: Balancer_States_Bus size=1; lightCalib data_store_memory; normalizedLight local single size=1; des_vel local single size=1; theta_ref local single size=1; forwardPWM local single size=1; turningPWM local single size=1; BT_status_out output single size=1; desired_phi local single size=1; phi0 local single size=1; turningPWML local; turningPWMR local

== stateflow chart see_saw_mario/see_saw_mario ==
  state see_saw_mode
    entry:
    desired_tail = single(1.6);
    BT_status_out = single(0);
    during:
    normalizedLight = processLight(sensors.light,lightCalib);
    PWM.tail = tail_controller(sensors.theta_T, desired_tail);
    DispVar(normalizedLight);
    state Pause
      entry:
      debugFlag = uint16(601);
    state light = processLight(rawLight,lightCalib) [function]
    state StandUp
      entry: debugFlag = uint16(602);
      initFlags.theta = single(1);
      initFlags.gyroReset = single(1);
      during:
      desired_tail = desired_tail + single(0.0008);
    state Balancing
      state SeesawLogic [parallel]
        settings: executionOrder=1
        state StationnaryBalance
          entry: debugFlag = uint16(603);
          desired_tail = single(0.5);
          initFlags.theta = single(0);
          initFlags.gyroReset = single(0);
          desired_states = balancerStates_Bus0;
        state Approach
          entry: debugFlag = uint16(604);
          during:
          turningPWM = lineTracker(single(-0.3), normalizedLight, single(1.3), sensors.battery);
          exit:
          turningPWM = single(0);
          state StartWalking
            entry:
            entry: debugFlag = uint16(605);
            des_vel = single(0.04);
            during:
            des_vel = des_vel+single(0.00024);
          state Walk
            entry: debugFlag = uint16(605);
          (default) -> StartWalking
          StartWalking -> Walk : [des_vel >= single(0.15)]
        state Seesaw
          state ControlledGoingUp
            entry:
            phi0 = states.phi;
            desired_phi = phi0;
            exit: turningPWM = single(0);
            state JumpOnIt
              entry:
              Speak;
              debugFlag = uint16(606);
              theta_ref = states.balancerStates.theta;
              des_vel = single(0.15);
            state GoingUP
              entry:
              debugFlag = uint16(607);
              des_vel = single(0.1);
              during:
              turningPWM = phiController(states.phi,desired_phi, sensors.battery)+...
              single(3)*lineTracker(single(0.15), normalizedLight, single(1), sensors.battery);
              exit:
              des_vel = single(0);
            state WaitForPrincess
              entry:
              debugFlag = uint16(608);
              BT_status_out = single(2);
              du:
              turningPWM = phiController(states.phi,desired_phi+single(0.2),sensors.battery);
            (default) -> JumpOnIt
            JumpOnIt -> GoingUP : [states.balancerStates.theta >= theta_ref+single(1.8)]
            GoingUP -> WaitForPrincess : [states.balancerStates.theta >= theta_ref + single(18)]
          state GoingDown
            during:
            turningPWM = single(-1.3)*lineTracker(single(0.5), normalizedLight, single(1.2), sensors.battery)+...
            single(0.5)*phiController(states.phi,desired_phi,sensors.battery);
            state GoingBack
              entry:
              debugFlag = uint16(609);
              des_vel = single(-0.06);
              exit:
              des_vel = single(-0.06);
            state WaitForPrincess2
              entry:
              debugFlag = uint16(610);
              BT_status_out = single(3);
              %during:turningPWM = phiController(states.phi,desired_phi,sensors.battery);
            state GetOff
              entry:
              debugFlag = uint16(611);
              des_vel = single(-0.1);
            state Pause3
              during:
              %turningPWM = phiController(states.phi,desired_phi,sensors.battery);
              des_vel = des_vel - single(0.00024);
            (default) -> GoingBack
            GoingBack -> WaitForPrincess2 : [states.balancerStates.theta <= theta_ref + single(12)]
            WaitForPrincess2 -> GetOff : [sensors.BT_status_in == single(103)]
            GetOff -> Pause3 : [states.balancerStates.theta <= theta_ref - single(7)]
          state GetOff1
            entry:
            debugFlag = uint16(6112);
            des_vel = single(-0.08);
            du:
            turningPWM = phiController(states.phi,desired_phi-single(0.2),sensors.battery);
          state FindingLine
            en:
            turningPWM = phiController(states.phi,desired_phi,sensors.battery);
            des_vel = single(0);
            state TurnAndBackup
              entry:
              debugFlag = uint16(612);
              BT_status_out = single(4);
              du:
              desired_phi = desired_phi - single(0.003);
              des_vel = single(0);
              turningPWM = phiController(states.phi,desired_phi,sensors.battery);
            state HuntLine
              entry: debugFlag = uint16(613)
              desired_phi = states.phi;
              theta_ref_2 = states.balancerStates.theta;
              du: turningPWM = phiController(states.phi,desired_phi,sensors.battery);
              state GoForward
                en:  des_vel= single(0.04);
              state BackUpB
                en: des_vel = single(-0.04)
              (default) -> GoForward
              BackUpB -> GoForward : [states.balancerStates.theta >= theta_ref_2 - single(3) ]
              GoForward -> BackUpB : [states.balancerStates.theta >= theta_ref_2 + single(3) ]
            state TurnAndBackup1
              entry:
              debugFlag = uint16(614);
              BT_status_out = single(4);
              des_vel = des_vel / single(2);
              du:
              desired_phi = desired_phi - single(0.003);
              turningPWM = phiController(states.phi,desired_phi,sensors.battery);
            state GoForwardUntilLine
              en:
              debugFlag = uint16(615)
              desired_phi = states.phi;
              du:
              turningPWM = lineTracker(single(0), normalizedLight, single(0.4), sensors.battery);
              des_vel= single(0.04);
            state BeginLineTrack
              en:
              debugFlag = uint16(616);
              des_vel =single(0.05);
              du:
              des_vel = des_vel+single(0.0004);
              turningPWM = lineTracker(single(0), normalizedLight, single(0.8), sensors.battery);
            state ConstantSpeedAlongLIne
              en:
              debugFlag = uint16(617);
              du:
              turningPWM = lineTracker(single(0), normalizedLight, single(1), sensors.battery);
            (default) -> TurnAndBackup
            TurnAndBackup -> HuntLine : [phi0-states.phi > single(1.6)]
            HuntLine -> TurnAndBackup1 : [normalizedLight >= single(0.5)]
            TurnAndBackup1 -> GoForwardUntilLine : [phi0-states.phi > single(3.2)]
            GoForwardUntilLine -> BeginLineTrack : after(3,sec)
            BeginLineTrack -> ConstantSpeedAlongLIne : [des_vel >= single(0.08)]
          state STOP
            en:
            des_vel = single(0);
          (default) -> ControlledGoingUp
          WaitForPrincess -> GoingDown : [sensors.BT_status_in == single(102)]
          Pause3 -> ? : [des_vel <= single(0)]
          GoingDown -> GetOff1 : [states.balancerStates.theta <= theta_ref ]
          GetOff1 -> FindingLine : [states.balancerStates.theta <= theta_ref - single(5)]
          ConstantSpeedAlongLIne -> STOP : [false] %[states.balancerStates.theta <= theta_ref - single(2)]
        state RaceDone
          entry: debugFlag = uint16(599);
          current_mode_status = OperationModeStatusEnum.SUCCESSFULLY_COMPLETED;
        (default) -> StationnaryBalance
        StationnaryBalance -> Approach : after(2,sec)
        Approach -> Seesaw : [states.balancerStates.theta_dot<single(-4)  && states.theta_dot_dot < single(-60) ]{BT_status_out = single(1);}
      state After [parallel]
        during:
        forwardPWM = balance_ctrl(states.balancerStates, des_vel ,sensors.battery)
        PWM.left = forwardPWM + turningPWM;
        PWM.right = forwardPWM - turningPWM;
        settings: executionOrder=2
    state DispVar(Var) [function]
    state cmd = phiController(phi,desiredPhi,battery) [function]
    state cmd = lineTracker(desiredLight,light,trackingPower,battery) [function]
    state Speak [function]
    state cmd = tail_controller(current,desired) [function]
    state cmd = balance_ctrl(balancerStates,desired_velocity,battery) [function]
    (default) -> Pause
    Pause -> StandUp
    StandUp -> Balancing : [desired_tail >=single(2.0) && sensors.theta_T >= single(2.0)]
  data: rawLight function_input single size=1; lightCalib function_input Bus: Light_Bus size=1; light function_output; Var function_input single size=1; cmd function_output; phi function_input single size=1; desiredPhi function_input single size=1; battery function_input double size=1; cmd function_output single size=1; desiredLight function_input single size=1; light function_input single size=1; trackingPower function_input single size=1; battery function_input double size=1; current function_input single size=1; desired function_input single size=1; cmd function_output single size=1; balancerStates function_input Bus: Balancer_States_Bus size=1; desired_velocity function_input single size=1; battery function_input double size=1; cmd function_output single size=1; states input Bus: States_Bus size=1; sensors input Bus: Sensors_Bus size=1; PWM output Bus: PWM_bus size=1; initFlags output Bus: Init_Bus size=1; debugFlag output uint16 size=1; desired_states local Bus: Balancer_States_Bus size=1; desired_tail local single size=1; current_mode_status data_store_memory; balancerStates_Bus0 parameter Bus: Balancer_States_Bus size=1; lightCalib data_store_memory; normalizedLight local single size=1; des_vel local single size=1; theta_ref local single size=1; forwardPWM local single size=1; turningPWM local single size=1; BT_status_out output single size=1; desired_phi local single size=1; phi0 local single size=1; theta_ref_2 local
